simulink model "Inverter3P_VoltageControl_PI_s"  (R2024a)
settings: Solver=ode23tb  StartTime=0.0  StopTime=0.6  RelTol=1e-4
undefined symbols (not defined in the file): Cf, kii, kiv, kpi, kpv, Lf, rL, Rload_dm
libraries: spsSeriesRLCBranchLib x12, spsCurrentMeasurementLib x6, spsIGBTDiodeLib x6, spsVoltageMeasurementLib x4, spsIdealSwitchLib x3, spsDCVoltageSourceLib x1, spsPower3phPhasorLib x1, sps_lib x1
Description:
  | Copyright 2008 The MathWorks(TM), Inc.
settings Model: Creator=patrice  LastModifiedBy=ducnv
settings SolverCC: AlgebraicLoopSolver=TrustRegion
settings DataIOCC: SaveFormat=Array  SignalLoggingSaveFormat=ModelDataLogs  ReturnWorkspaceOutputs=off  SignalLoggingName=sigsOut
settings OptimizationCC: BlockReduction=off  BooleanDataType=off  ExpressionDepthLimit=2147483647  InitFltsAndDblsToZero=on  EfficientMapNaN2IntZero=off  LifeSpan=inf
settings DebuggingCC: UnderspecifiedInitializationDetection=Classic  MergeDetectMultiDrivingBlocksExec=none  CheckExecutionContextPreStartOutputMsg=on  SignalResolutionControl=TryResolveAllWithWarning  MultiTaskDSMMsg=warning  MultiTaskCondExecSysMsg=none  SigSpecEnsureSampleTimeMsg=none  FcnCallInpInsideContextMsg=warning  UnconnectedInputMsg=warning  UnconnectedOutputMsg=warning  UnconnectedLineMsg=warning  StateNameClashWarn=warning  SFUnexpectedBacktrackingDiag=warning  SFNoUnconditionalDefaultTransitionDiag=warning  SFExecutionAtInitializationDiag=none  ArithmeticOperatorsInVariantConditions=warning
settings HardwareCC: ProdBitPerPointer=32  ProdBitPerSizeT=32  ProdBitPerPtrDiffT=32  ProdLargestAtomicFloat=None  ProdIntDivRoundTo=Undefined  ProdEndianess=Unspecified  ProdWordSize=32  ProdHWDeviceType=32-bit Generic  TargetUnknown=on
settings ModelReferenceCC: PropagateSignalLabelsOutOfModel=off
settings SFSimCC: SimUseLocalCustomCode=off  CustomCodeUndefinedFunction=UseInterfaceOnly
settings RTWCC: RTWUseLocalCustomCode=off  GPUComputeCapability=3.5
settings CodeAppCC: StateflowObjectComments=on
settings GRTTargetCC: TargetLangStandard=C89/C90 (ANSI)  CombineOutputUpdateFcns=off  GRTInterface=on
settings ConfigComp: CovMetricSettings=dw  CovSaveCumulativeToWorkspaceVar=on  CovSaveSingleToWorkspaceVar=on  CovExternalEMLEnable=off
settings SimscapeCC: SimscapeNormalizeSystem=off

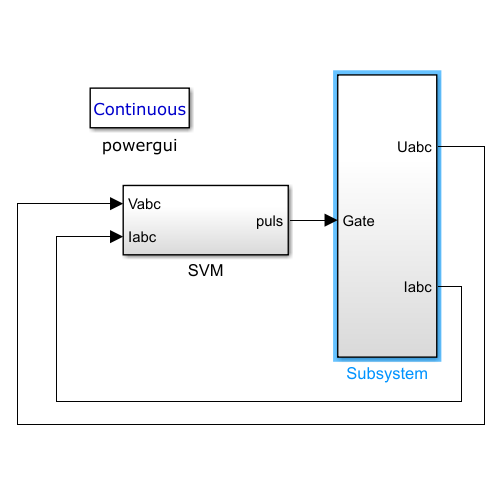
[thumbnail: Simulink's stored preview of the top-level diagram]
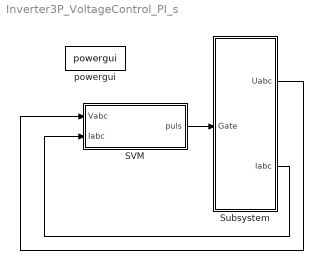
== system Inverter3P_VoltageControl_PI_s ==
  SVM : Subsystem
  Subsystem : Subsystem
  powergui : sps_lib/powergui  SimulationMode=Continuous  SampleTime=200e-6  frequency=60  Iterations=50  frequencyindice=0  Pbase=100e6  ErrMax=1e-4  UnitsV=kV  UnitsW=MW  buscounter=0  FunctionMessages=off  echomessages=off  EnableUseOfTLC=off  CurrentSourceSwitches=on  DisableSnubberDevices=off  DisableRonSwitches=off  DisableVfSwitches=off  DisplayEquations=off  AutomaticDiscreteSolvers=off  SolverType=Tustin  Interpol=off  ExternalGateDelay=off  methode=off  Ts=0  x0status=blocks  SPID=off  SwTol=0  HookPort=off  NonlinearTolerance=1e-4  nMaxIteration=100  ContinueOnMaxIteration=off  RestoreLinks=warning  ResistiveCurrentMeasurement=off  Frange=[0:2:500]  Ylog=off  Xlog=on  ShowGrid=off  save=off  variable=ZData  structure=ScopeData  ZoomFFT=off  StartTime=0.02  cycles=2  DisplayStyle=1  fundamental=50  FreqAxis=on  MaxFrequency=20000  frequencyindicesteady=1  RmsSteady=1  display=off
  wires:
  SVM/1(puls) -> Subsystem/1(Gate)
  Subsystem/2(Iabc) -> SVM/2(Iabc)
  Subsystem/1(Uabc) -> SVM/1(Vabc)

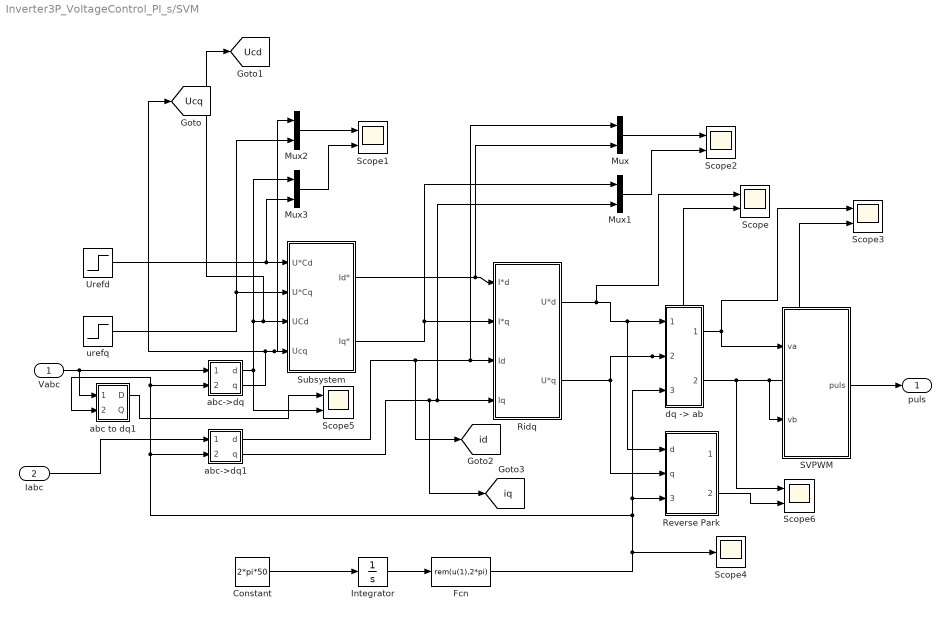
== system Inverter3P_VoltageControl_PI_s/SVM ==
  Vabc : Inport
  Iabc : Inport  Port=2
  Constant : Constant  Value=2*pi*50
  Fcn : Fcn  Expr=rem(u(1),2*pi)
  Integrator : Integrator
  Mux{,1..3} (4 alike) : Mux  Inputs=2
  Reverse Park : Subsystem
  Ridq : Subsystem
  SVPWM : Subsystem
  Scope{,1..3,5..6} (6 alike) : Scope  NumInputPorts=2
  Scope4 : Scope
  Subsystem : Subsystem
  Urefd : Step  Time=0  After=100  SampleTime=0
  abc to dq1 : Subsystem
  abc->dq : Subsystem  AncestorBlock=plecslib_extras/Transformations/3ph->RRF  mask(Transformation 3ph->RRF){}
      mask help:
      | Transforms a three-phase signal into a two-dimensional vector in a rotating reference frame. The rotation angle in radians of the rotating reference frame is determined by the second input:
      | [a b c], phi -> [d q]
      mask Help: web(['file://' plecsdoc '/abc2dq.html'])
      mask Display: plot([0 100],[0 100], [0.5 3 4 4 5 4 3 1 0 0 1 4]*4,[7 7 6 3 2 3 2 2 3 4 5 5]*4+62, [0 1 3 4 4 3 1 0 0 0]*4+24,[6 7 7 6 3 2 2 3 2 10]*4+62, [4 3 1 0 0 1 3 4]*4+48,[6 7 7 6 3 2 2 3]*4+62, [4 3 1 0 0 1 3 4 4 4]*4+52,[6 7 7 6 3 2 2 3 2 10]*4+5, [4 3 1 0 0 1 3 4 4 4]*4+76,[3 2 2 3 6 7 7 6 7 0]*4+5 )
  abc->dq1 : Subsystem  AncestorBlock=plecslib_extras/Transformations/3ph->RRF  mask(Transformation 3ph->RRF){}
      mask help:
      | Transforms a three-phase signal into a two-dimensional vector in a rotating reference frame. The rotation angle in radians of the rotating reference frame is determined by the second input:
      | [a b c], phi -> [d q]
      mask Help: web(['file://' plecsdoc '/abc2dq.html'])
      mask Display: plot([0 100],[0 100], [0.5 3 4 4 5 4 3 1 0 0 1 4]*4,[7 7 6 3 2 3 2 2 3 4 5 5]*4+62, [0 1 3 4 4 3 1 0 0 0]*4+24,[6 7 7 6 3 2 2 3 2 10]*4+62, [4 3 1 0 0 1 3 4]*4+48,[6 7 7 6 3 2 2 3]*4+62, [4 3 1 0 0 1 3 4 4 4]*4+52,[6 7 7 6 3 2 2 3 2 10]*4+5, [4 3 1 0 0 1 3 4 4 4]*4+76,[3 2 2 3 6 7 7 6 7 0]*4+5 )
  "dq -> ab" : Subsystem  mask(Coordinate converter){}
      mask help: The block converts 2 voltage (or rotor current , magnetic flux...) components which locate in rotor flux coordinate into 2 components located in fixed stator coordinate.The real axises of two coordinate locate askew each other an angle specified by the third input . The block has no parameters.
      mask Display:
      | plot([0 1],[0 1]);
      | text(0.3,0.7,'dq');text(0.7,0.4,'ab');
  urefq : Step  Time=0  After=sqrt(((220*sqrt(2))^2)-100^2)  SampleTime=0
  puls : Outport
  tag scope: Ucd=global, Ucq=global, id=global, iq=global
  wires:
  "dq -> ab"/1(Out1) -> Scope3/1, SVPWM/1(va)
  "dq -> ab"/2(Out2) -> Scope6/1, Scope3/2, SVPWM/2(vb)
  SVPWM/1(puls) -> puls/1
  Constant/1 -> Integrator/1
  Integrator/1 -> Fcn/1
  Ridq/1(U*d) -> Scope/1, Reverse Park/1(d), "dq -> ab"/1(In1)
  Ridq/2(U*q) -> Reverse Park/2(q), Scope/2, "dq -> ab"/2(In2)
  Urefd/1 -> Mux3/2, Subsystem/1(U*Cd)
  urefq/1 -> Mux2/2, Subsystem/2(U*Cq)
  abc->dq/1(d) -> Scope5/2, Mux3/1, [Ucd], Subsystem/3(UCd)
  abc->dq/2(q) -> [Ucq], Mux2/1, Subsystem/4(Ucq)
  abc->dq1/1(d) -> [id], Mux/1, Ridq/3(Id)
  abc->dq1/2(q) -> [iq], Mux1/2, Ridq/4(Iq)
  Vabc/1 -> abc to dq1/1(abc), abc->dq/1(abc)
  Iabc/1 -> abc->dq1/1(abc)
  Mux/1 -> Scope2/1
  Mux1/1 -> Scope2/2
  Mux2/1 -> Scope1/1
  Mux3/1 -> Scope1/2
  Fcn/1 -> Scope4/1, Reverse Park/3(Theta), "dq -> ab"/3(In3), abc->dq1/2(phi), abc to dq1/2(Theta), abc->dq/2(phi)
  abc to dq1/1(D) -> Scope5/1
  Reverse Park/2(Beta) -> Scope6/2
  Subsystem/1(Id*) -> Mux/2, Ridq/1(I*d)
  Subsystem/2(Iq*) -> Mux1/1, Ridq/2(I*q)

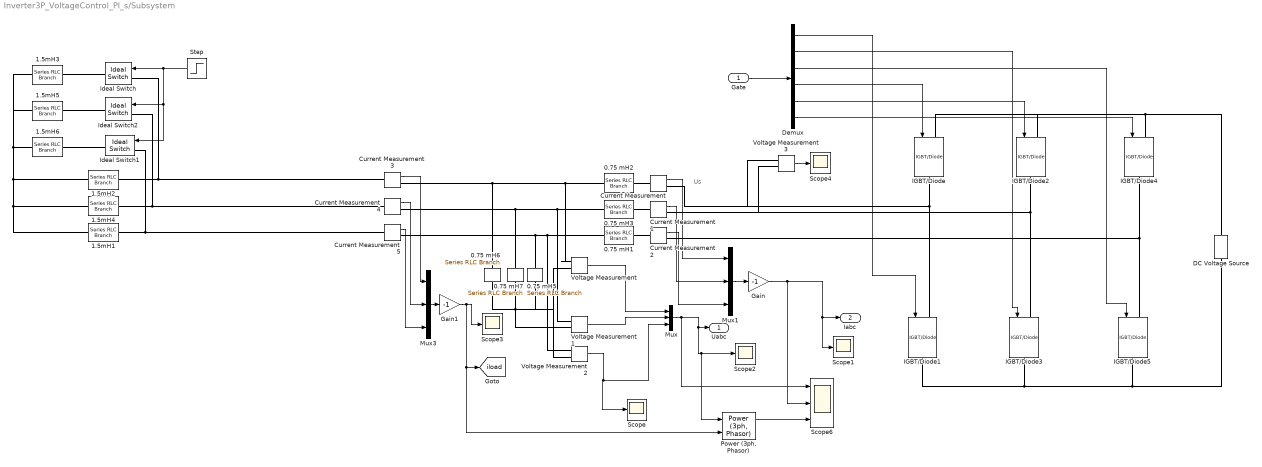
== system Inverter3P_VoltageControl_PI_s/Subsystem ==
  note: Us
  Gate : Inport
  0.75 mH1 : spsSeriesRLCBranchLib/Series RLC Branch  LConnTagsString=__new0  RConnTagsString=__new0  BranchType=RL  Resistance=rL  Inductance=Lf  SetiL0=off  InitialCurrent=0  Capacitance=1.0  Setx0=off  InitialVoltage=0  Measurements=None
  0.75 mH2 : spsSeriesRLCBranchLib/Series RLC Branch  LConnTagsString=__new0  RConnTagsString=__new0  BranchType=RL  Resistance=rL  Inductance=Lf  SetiL0=off  InitialCurrent=0  Capacitance=1.0  Setx0=off  InitialVoltage=0  Measurements=None
  0.75 mH3 : spsSeriesRLCBranchLib/Series RLC Branch  LConnTagsString=__new0  RConnTagsString=__new0  BranchType=RL  Resistance=rL  Inductance=Lf  SetiL0=off  InitialCurrent=0  Capacitance=1.0  Setx0=off  InitialVoltage=0  Measurements=None
  0.75 mH5 : spsSeriesRLCBranchLib/Series RLC Branch  LConnTagsString=__new0  RConnTagsString=__new0  BranchType=C  Resistance=1.0  Inductance=0.75e-3  SetiL0=off  InitialCurrent=0  Capacitance=Cf  Setx0=off  InitialVoltage=0  Measurements=None
  0.75 mH6 : spsSeriesRLCBranchLib/Series RLC Branch  LConnTagsString=__new0  RConnTagsString=__new0  BranchType=C  Resistance=1.0  Inductance=0.75e-3  SetiL0=off  InitialCurrent=0  Capacitance=Cf  Setx0=off  InitialVoltage=0  Measurements=None
  0.75 mH7 : spsSeriesRLCBranchLib/Series RLC Branch  LConnTagsString=__new0  RConnTagsString=__new0  BranchType=C  Resistance=1.0  Inductance=0.75e-3  SetiL0=off  InitialCurrent=0  Capacitance=Cf  Setx0=off  InitialVoltage=0  Measurements=None
  1.5mH{1..6} (6 alike) : spsSeriesRLCBranchLib/Series RLC Branch  LConnTagsString=__new0  RConnTagsString=__new0  BranchType=R  Resistance=Rload_dm*1.5  Inductance=2e-3  SetiL0=off  InitialCurrent=0  Capacitance=1.0  Setx0=off  InitialVoltage=0  Measurements=None
  Current Measurement{,1..5} (6 alike) : spsCurrentMeasurementLib/Current Measurement  PhasorSimulation=off  OutputType=Complex  PSBequivalent=0
  DC Voltage Source : spsDCVoltageSourceLib/DC Voltage Source  Amplitude=600  Measurements=None
  Demux : Demux  Outputs=6
  Gain : Gain  Gain=-1
  Gain1 : Gain  Gain=-1
  IGBT/Diode{,1..5} (6 alike) : spsIGBTDiodeLib/IGBT//Diode  Ron=1e-3  Rs=1e5  Cs=inf  Measurements=off
  Ideal Switch : spsIdealSwitchLib/Ideal Switch  Ron=0.001  Lon=0  IC=0  Rs=1e5  Cs=inf  Measurements=off
  Ideal Switch1 : spsIdealSwitchLib/Ideal Switch  Ron=0.001  Lon=0  IC=0  Rs=1e5  Cs=inf  Measurements=off
  Ideal Switch2 : spsIdealSwitchLib/Ideal Switch  Ron=0.001  Lon=0  IC=0  Rs=1e5  Cs=inf  Measurements=off
  Mux : Mux  Inputs=3
  Mux1 : Mux  Inputs=3
  Mux3 : Mux  Inputs=3
  "Power (3ph, Phasor)" : spsPower3phPhasorLib/Power (3ph, Phasor)
      settings: LibrarySourceBlock=|
      | sps_lib/Sensors and Measurements/Power
      | (3ph, Phasor)
  Scope{,1..4} (5 alike) : Scope
  Scope6 : Scope  NumInputPorts=3
  Step : Step  Time=0.3  SampleTime=0
  Voltage Measurement{,1..3} (4 alike) : spsVoltageMeasurementLib/Voltage Measurement  PhasorSimulation=off  OutputType=Complex  PSBequivalent=0
  Uabc : Outport
  Iabc : Outport  Port=2
  tag scope: iload=global
  wires:
  Gate/1 -> Demux/1
  Mux/1 -> Scope6/1, "Power (3ph, Phasor)"/1, Scope2/1, Uabc/1
  Mux1/1 -> Gain/1
  Gain/1 -> Scope6/2, Scope1/1, Iabc/1
  Voltage Measurement/1 -> Mux/1
  Voltage Measurement1/1 -> Mux/2
  Voltage Measurement2/1 -> Scope/1, Mux/3
  Current Measurement/1 -> Mux1/1
  Current Measurement1/1 -> Mux1/2
  Current Measurement2/1 -> Mux1/3
  Mux3/1 -> Gain1/1
  Gain1/1 -> [iload], "Power (3ph, Phasor)"/2, Scope3/1
  Current Measurement3/1 -> Mux3/1
  Current Measurement4/1 -> Mux3/2
  Current Measurement5/1 -> Mux3/3
  Voltage Measurement3/1 -> Scope4/1
  Demux/1 -> IGBT/Diode1/1
  Demux/2 -> IGBT/Diode3/1
  Demux/3 -> IGBT/Diode5/1
  Demux/4 -> IGBT/Diode/1
  Demux/5 -> IGBT/Diode2/1
  Demux/6 -> IGBT/Diode4/1
  Step/1 -> Ideal Switch1/1, Ideal Switch2/1, Ideal Switch/1
  "Power (3ph, Phasor)"/1 -> Scope6/3
  connections:
  IGBT/Diode2/LConn1 -- IGBT/Diode/LConn1 -- IGBT/Diode4/LConn1 -- DC Voltage Source/RConn1
  IGBT/Diode5/RConn1 -- IGBT/Diode1/RConn1 -- IGBT/Diode3/RConn1 -- DC Voltage Source/LConn1
  IGBT/Diode2/RConn1 -- Voltage Measurement3/LConn2 -- Current Measurement1/RConn1 -- IGBT/Diode3/LConn1
  IGBT/Diode5/LConn1 -- Current Measurement2/RConn1 -- IGBT/Diode4/RConn1
  IGBT/Diode/RConn1 -- Voltage Measurement3/LConn1 -- Current Measurement/RConn1 -- IGBT/Diode1/LConn1
  0.75 mH5/RConn1 -- Current Measurement5/RConn1 -- 0.75 mH1/LConn1 -- Voltage Measurement2/LConn1
  0.75 mH7/RConn1 -- Current Measurement4/RConn1 -- 0.75 mH3/LConn1 -- Voltage Measurement1/LConn1
  0.75 mH6/RConn1 -- Current Measurement3/RConn1 -- Voltage Measurement/LConn1 -- 0.75 mH2/LConn1
  0.75 mH2/RConn1 -- Current Measurement/LConn1
  0.75 mH3/RConn1 -- Current Measurement1/LConn1
  0.75 mH1/RConn1 -- Current Measurement2/LConn1
  0.75 mH6/LConn1 -- Voltage Measurement/LConn2 -- Voltage Measurement2/LConn2 -- Voltage Measurement1/LConn2 -- 0.75 mH7/LConn1 -- 0.75 mH5/LConn1
  Ideal Switch/LConn1 -- Current Measurement3/LConn1 -- 1.5mH2/LConn1
  Current Measurement5/LConn1 -- Ideal Switch1/LConn1 -- 1.5mH1/LConn1
  Current Measurement4/LConn1 -- Ideal Switch2/LConn1 -- 1.5mH4/LConn1
  1.5mH2/RConn1 -- 1.5mH3/RConn1 -- 1.5mH5/RConn1 -- 1.5mH6/RConn1 -- 1.5mH1/RConn1 -- 1.5mH4/RConn1
  1.5mH6/LConn1 -- Ideal Switch1/RConn1
  1.5mH5/LConn1 -- Ideal Switch2/RConn1
  1.5mH3/LConn1 -- Ideal Switch/RConn1

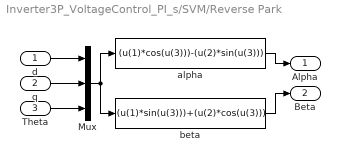
== system Inverter3P_VoltageControl_PI_s/SVM/Reverse Park ==
  d : Inport
  q : Inport  Port=2
  Theta : Inport  Port=3
  Mux : Mux  Inputs=3
  alpha : Fcn  Expr=(u(1)*cos(u(3)))-(u(2)*sin(u(3)))
  beta : Fcn  Expr=(u(1)*sin(u(3)))+(u(2)*cos(u(3)))
  Alpha : Outport  VectorParamsAs1DForOutWhenUnconnected=off
  Beta : Outport  Port=2  VectorParamsAs1DForOutWhenUnconnected=off
  wires:
  alpha/1 -> Alpha/1
  beta/1 -> Beta/1
  Mux/1 -> beta/1, alpha/1
  d/1 -> Mux/1
  q/1 -> Mux/2
  Theta/1 -> Mux/3

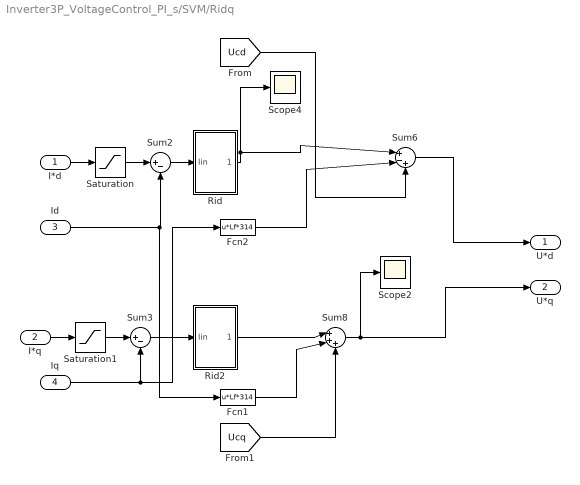
== system Inverter3P_VoltageControl_PI_s/SVM/Ridq ==
  I*d : Inport
  I*q : Inport  Port=2
  Id : Inport  Port=3
  Iq : Inport  Port=4
  Fcn1 : Fcn  Expr=u*Lf*314
  Fcn2 : Fcn  Expr=u*Lf*314
  Rid : Subsystem
  Rid2 : Subsystem
  Saturation : Saturate  UpperLimit=15.15*sqrt(2)
  Saturation1 : Saturate  UpperLimit=15.15*sqrt(2)
  Scope2 : Scope
  Scope4 : Scope
  Sum2 : Sum  Inputs=|+-
  Sum3 : Sum  Inputs=|+-
  Sum6 : Sum  Inputs=|+-+
  Sum8 : Sum  Inputs=|+++
  U*d : Outport
  U*q : Outport  Port=2
  wires:
  Id/1 -> Fcn1/1, Sum2/2
  I*d/1 -> Saturation/1
  I*q/1 -> Saturation1/1
  Fcn1/1 -> Sum8/2
  Fcn2/1 -> Sum6/2
  Sum3/1 -> Rid2/1(Iin)
  Sum2/1 -> Rid/1(Iin)
  Iq/1 -> Fcn2/1, Sum3/2
  Sum8/1 -> Scope2/1, U*q/1
  Sum6/1 -> U*d/1
  [Ucq] -> Sum8/3
  [Ucd] -> Sum6/3
  Rid/1(dUL) -> Sum6/1, Scope4/1
  Rid2/1(dUL) -> Sum8/1
  Saturation/1 -> Sum2/1
  Saturation1/1 -> Sum3/1

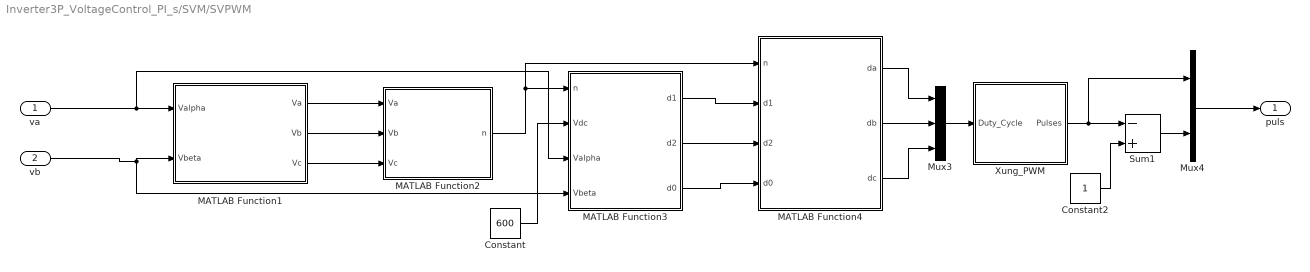
== system Inverter3P_VoltageControl_PI_s/SVM/SVPWM ==
  va : Inport
  vb : Inport  Port=2
  Constant : Constant  Value=600
  Constant2 : Constant
  MATLAB Function1 : MATLAB Function  TreatAsAtomicUnit=on
  MATLAB Function2 : MATLAB Function  TreatAsAtomicUnit=on
  MATLAB Function3 : MATLAB Function  TreatAsAtomicUnit=on
  MATLAB Function4 : MATLAB Function  TreatAsAtomicUnit=on
  Mux3 : Mux  Inputs=3
  Mux4 : Mux  Inputs=2
  Sum1 : Sum  Inputs=-+
  Xung_PWM : Subsystem
  puls : Outport
  wires:
  Constant/1 -> MATLAB Function3/2(Vdc)
  MATLAB Function1/3(Vc) -> MATLAB Function2/3(Vc)
  MATLAB Function1/2(Vb) -> MATLAB Function2/2(Vb)
  Mux4/1 -> puls/1
  Sum1/1 -> Mux4/2
  Xung_PWM/1(Pulses) -> Mux4/1, Sum1/1
  MATLAB Function2/1(n) -> MATLAB Function4/1(n), MATLAB Function3/1(n)
  Mux3/1 -> Xung_PWM/1(Duty_Cycle)
  vb/1 -> MATLAB Function3/4(Vbeta), MATLAB Function1/2(Vbeta)
  MATLAB Function3/3(d0) -> MATLAB Function4/4(d0)
  MATLAB Function3/1(d1) -> MATLAB Function4/2(d1)
  MATLAB Function4/1(da) -> Mux3/1
  MATLAB Function1/1(Va) -> MATLAB Function2/1(Va)
  MATLAB Function4/3(dc) -> Mux3/3
  MATLAB Function3/2(d2) -> MATLAB Function4/3(d2)
  MATLAB Function4/2(db) -> Mux3/2
  va/1 -> MATLAB Function3/3(Valpha), MATLAB Function1/1(Valpha)
  Constant2/1 -> Sum1/2

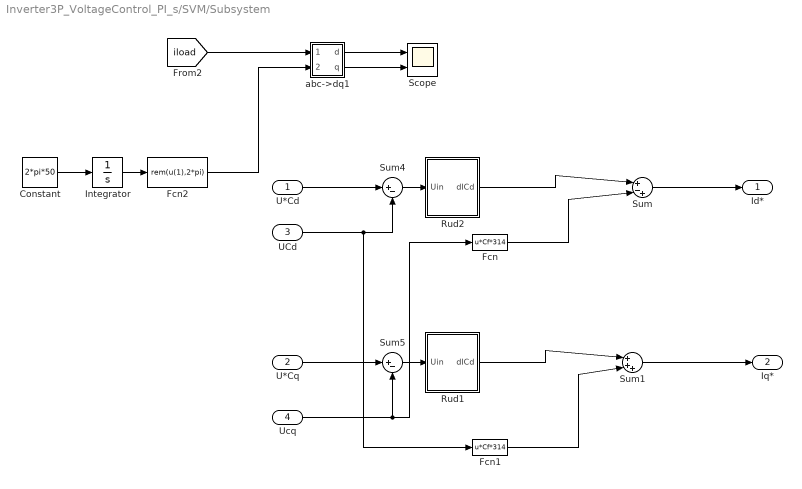
== system Inverter3P_VoltageControl_PI_s/SVM/Subsystem ==
  U*Cd : Inport
  U*Cq : Inport  Port=2
  UCd : Inport  Port=3
  Ucq : Inport  Port=4
  Constant : Constant  Value=2*pi*50
  Fcn : Fcn  Expr=u*Cf*314
  Fcn1 : Fcn  Expr=u*Cf*314
  Fcn2 : Fcn  Expr=rem(u(1),2*pi)
  Integrator : Integrator
  Rud1 : Subsystem
  Rud2 : Subsystem
  Scope : Scope  NumInputPorts=2
  Sum : Sum  Inputs=|+-+
  Sum1 : Sum  Inputs=|+++
  Sum4 : Sum  Inputs=|+-
  Sum5 : Sum  Inputs=|+-
  abc->dq1 : Subsystem  AncestorBlock=plecslib_extras/Transformations/3ph->RRF  mask(Transformation 3ph->RRF){}
      mask help:
      | Transforms a three-phase signal into a two-dimensional vector in a rotating reference frame. The rotation angle in radians of the rotating reference frame is determined by the second input:
      | [a b c], phi -> [d q]
      mask Help: web(['file://' plecsdoc '/abc2dq.html'])
      mask Display: plot([0 100],[0 100], [0.5 3 4 4 5 4 3 1 0 0 1 4]*4,[7 7 6 3 2 3 2 2 3 4 5 5]*4+62, [0 1 3 4 4 3 1 0 0 0]*4+24,[6 7 7 6 3 2 2 3 2 10]*4+62, [4 3 1 0 0 1 3 4]*4+48,[6 7 7 6 3 2 2 3]*4+62, [4 3 1 0 0 1 3 4 4 4]*4+52,[6 7 7 6 3 2 2 3 2 10]*4+5, [4 3 1 0 0 1 3 4 4 4]*4+76,[3 2 2 3 6 7 7 6 7 0]*4+5 )
  Id* : Outport
  Iq* : Outport  Port=2
  wires:
  Sum/1 -> Id*/1
  Sum1/1 -> Iq*/1
  UCd/1 -> Fcn1/1, Sum4/2
  Ucq/1 -> Fcn/1, Sum5/2
  U*Cq/1 -> Sum5/1
  Rud1/1(dICd) -> Sum1/1
  Rud2/1(dICd) -> Sum/1
  Sum4/1 -> Rud2/1(Uin)
  Fcn1/1 -> Sum1/2
  Sum5/1 -> Rud1/1(Uin)
  Fcn/1 -> Sum/2
  U*Cd/1 -> Sum4/1
  [iload] -> abc->dq1/1(abc)
  Integrator/1 -> Fcn2/1
  Constant/1 -> Integrator/1
  Fcn2/1 -> abc->dq1/2(phi)
  abc->dq1/1(d) -> Scope/1
  abc->dq1/2(q) -> Scope/2

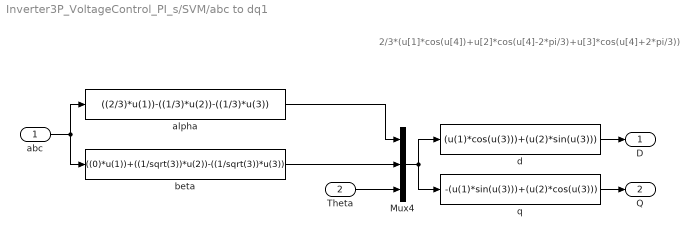
== system Inverter3P_VoltageControl_PI_s/SVM/abc to dq1 ==
  note: 2/3*(u[1]*cos(u[4])+u[2]*cos(u[4]-2*pi/3)+u[3]*cos(u[4]+2*pi/3))
  abc : Inport
  Theta : Inport  Port=2
  Mux4 : Mux  Inputs=3
  alpha : Fcn  Expr=((2/3)*u(1))-((1/3)*u(2))-((1/3)*u(3))
  beta : Fcn  Expr=((0)*u(1))+((1/sqrt(3))*u(2))-((1/sqrt(3))*u(3))
  d : Fcn  Expr=(u(1)*cos(u(3)))+(u(2)*sin(u(3)))
  q : Fcn  Expr=-(u(1)*sin(u(3)))+(u(2)*cos(u(3)))
  D : Outport  VectorParamsAs1DForOutWhenUnconnected=off
  Q : Outport  Port=2  VectorParamsAs1DForOutWhenUnconnected=off
  wires:
  Theta/1 -> Mux4/3
  q/1 -> Q/1
  alpha/1 -> Mux4/1
  d/1 -> D/1
  beta/1 -> Mux4/2
  abc/1 -> alpha/1, beta/1
  Mux4/1 -> d/1, q/1

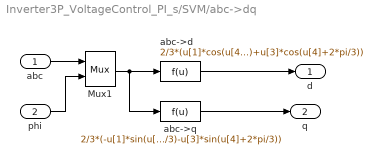
== system Inverter3P_VoltageControl_PI_s/SVM/abc->dq ==
  abc : Inport  PortDimensions=3
  phi : Inport  Port=2  PortDimensions=1
  Mux1 : Mux  Inputs=2
  abc->d : Fcn  Expr=2/3*(u[1]*cos(u[4])+u[2]*cos(u[4]-2*pi/3)+u[3]*cos(u[4]+2*pi/3))
  abc->q : Fcn  Expr=2/3*(-u[1]*sin(u[4])-u[2]*sin(u[4]-2*pi/3)-u[3]*sin(u[4]+2*pi/3))
  d : Outport
  q : Outport  Port=2
  wires:
  Mux1/1 -> abc->d/1, abc->q/1
  abc->q/1 -> q/1
  abc->d/1 -> d/1
  abc/1 -> Mux1/1
  phi/1 -> Mux1/2

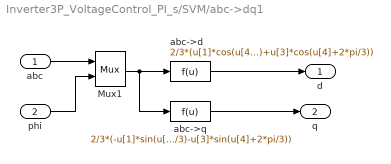
== system Inverter3P_VoltageControl_PI_s/SVM/abc->dq1 ==
  abc : Inport  PortDimensions=3
  phi : Inport  Port=2  PortDimensions=1
  Mux1 : Mux  Inputs=2
  abc->d : Fcn  Expr=2/3*(u[1]*cos(u[4])+u[2]*cos(u[4]-2*pi/3)+u[3]*cos(u[4]+2*pi/3))
  abc->q : Fcn  Expr=2/3*(-u[1]*sin(u[4])-u[2]*sin(u[4]-2*pi/3)-u[3]*sin(u[4]+2*pi/3))
  d : Outport
  q : Outport  Port=2
  wires:
  phi/1 -> Mux1/2
  abc/1 -> Mux1/1
  abc->d/1 -> d/1
  abc->q/1 -> q/1
  Mux1/1 -> abc->q/1, abc->d/1

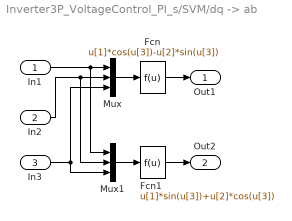
== system Inverter3P_VoltageControl_PI_s/SVM/dq -> ab ==
  In1 : Inport
  In2 : Inport  Port=2
  In3 : Inport  Port=3
  Fcn : Fcn  Expr=u[1]*cos(u[3])-u[2]*sin(u[3])
  Fcn1 : Fcn  Expr=u[1]*sin(u[3])+u[2]*cos(u[3])
  Mux : Mux  Inputs=3
  Mux1 : Mux  Inputs=3
  Out1 : Outport  InitialOutput=0
  Out2 : Outport  Port=2  InitialOutput=0
  wires:
  In1/1 -> Mux/1, Mux1/1
  In2/1 -> Mux/2, Mux1/2
  In3/1 -> Mux/3, Mux1/3
  Mux/1 -> Fcn/1
  Mux1/1 -> Fcn1/1
  Fcn/1 -> Out1/1
  Fcn1/1 -> Out2/1

== system Inverter3P_VoltageControl_PI_s/SVM/Ridq/Rid ==
  Iin : Inport
  Gain : Gain  Gain=kii
  Gain1 : Gain  Gain=kpi
  Integrator : Integrator
  Sum : Sum  Inputs=|++
  dUL : Outport
  wires:
  Sum/1 -> dUL/1
  Integrator/1 -> Sum/2
  Gain1/1 -> Sum/1
  Gain/1 -> Integrator/1
  Iin/1 -> Gain/1, Gain1/1

== system Inverter3P_VoltageControl_PI_s/SVM/Ridq/Rid2 ==
  Iin : Inport
  Gain : Gain  Gain=kii
  Gain1 : Gain  Gain=kpi
  Integrator : Integrator
  Sum : Sum  Inputs=|++
  dUL : Outport
  wires:
  Sum/1 -> dUL/1
  Integrator/1 -> Sum/2
  Gain1/1 -> Sum/1
  Gain/1 -> Integrator/1
  Iin/1 -> Gain/1, Gain1/1

== system Inverter3P_VoltageControl_PI_s/SVM/SVPWM/Xung_PWM ==
  Duty_Cycle : Inport
  Relay : Relay
  Sawtooth : Subsystem
  Scope : Scope
  Sum4 : Sum  Inputs=-+|  InputSameDT=on  SaturateOnIntegerOverflow=on  OutDataTypeStr=Inherit: Same as first input
  Pulses : Outport  VectorParamsAs1DForOutWhenUnconnected=off
  wires:
  Sum4/1 -> Relay/1
  Duty_Cycle/1 -> Sum4/2
  Sawtooth/1(Pulses) -> Scope/1, Sum4/1
  Relay/1 -> Pulses/1

== system Inverter3P_VoltageControl_PI_s/SVM/Subsystem/Rud1 ==
  Uin : Inport
  Gain : Gain  Gain=kiv
  Gain1 : Gain  Gain=kpv
  Integrator : Integrator
  Sum : Sum  Inputs=|++
  dICd : Outport
  wires:
  Integrator/1 -> Sum/2
  Uin/1 -> Gain1/1, Gain/1
  Gain1/1 -> Sum/1
  Gain/1 -> Integrator/1
  Sum/1 -> dICd/1

== system Inverter3P_VoltageControl_PI_s/SVM/Subsystem/Rud2 ==
  Uin : Inport
  Gain : Gain  Gain=kiv
  Gain1 : Gain  Gain=kpv
  Integrator : Integrator
  Sum : Sum  Inputs=|++
  dICd : Outport
  wires:
  Integrator/1 -> Sum/2
  Uin/1 -> Gain1/1, Gain/1
  Gain1/1 -> Sum/1
  Gain/1 -> Integrator/1
  Sum/1 -> dICd/1

== system Inverter3P_VoltageControl_PI_s/SVM/Subsystem/abc->dq1 ==
  abc : Inport  PortDimensions=3
  phi : Inport  Port=2  PortDimensions=1
  Mux1 : Mux  Inputs=2
  abc->d : Fcn  Expr=2/3*(u[1]*cos(u[4])+u[2]*cos(u[4]-2*pi/3)+u[3]*cos(u[4]+2*pi/3))
  abc->q : Fcn  Expr=2/3*(-u[1]*sin(u[4])-u[2]*sin(u[4]-2*pi/3)-u[3]*sin(u[4]+2*pi/3))
  d : Outport
  q : Outport  Port=2
  wires:
  phi/1 -> Mux1/2
  abc/1 -> Mux1/1
  abc->d/1 -> d/1
  abc->q/1 -> q/1
  Mux1/1 -> abc->q/1, abc->d/1

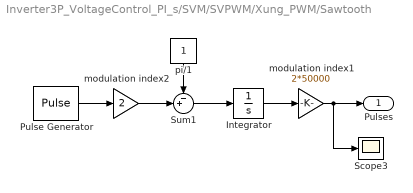
== system Inverter3P_VoltageControl_PI_s/SVM/SVPWM/Xung_PWM/Sawtooth ==
  Integrator : Integrator
  Pulse Generator : DiscretePulseGenerator  PulseType=Time based  Period=1/50000  PulseWidth=50
  Scope3 : Scope
  Sum1 : Sum  Inputs=-+|  InputSameDT=on  SaturateOnIntegerOverflow=on  OutDataTypeStr=Inherit: Same as first input
  modulation index1 : Gain  Gain=2*50000  SaturateOnIntegerOverflow=on  OutDataTypeStr=Inherit: Same as input  ParamDataTypeStr=Inherit: Same as input
  modulation index2 : Gain  Gain=2  SaturateOnIntegerOverflow=on  OutDataTypeStr=Inherit: Same as input  ParamDataTypeStr=Inherit: Same as input
  pi/1 : Constant
  Pulses : Outport  VectorParamsAs1DForOutWhenUnconnected=off
  wires:
  Pulse Generator/1 -> modulation index2/1
  Integrator/1 -> modulation index1/1
  modulation index1/1 -> Pulses/1, Scope3/1
  Sum1/1 -> Integrator/1
  modulation index2/1 -> Sum1/2
  pi/1/1 -> Sum1/1

== matlab function Inverter3P_VoltageControl_PI_s/SVM/SVPWM/MATLAB Function1 ==
  data: Valpha input; Va output; Vbeta input; Vb output; Vc output
function [Va,Vb,Vc] = Rev_Clark(Valpha,Vbeta)
Va = Valpha;
Vb = -Valpha/2 + sqrt(3)*Vbeta/2;
Vc = -Valpha/2 - sqrt(3)*Vbeta/2;

== matlab function Inverter3P_VoltageControl_PI_s/SVM/SVPWM/MATLAB Function2 ==
  data: Va input; n output; Vb input; Vc input
function n = Sector(Va,Vb,Vc)
n = 0;
if (Va >= Vb)
    if(Vb >= Vc)
        n = 1;
    else
        if (Vc >= Va)
            n = 5;
        else
            n = 6;
        end
    end
else
    if (Vb < Vc)
        n = 4;
    else
        if (Vc < Va)
            n = 2;
        else
            n = 3;
        end
    end
end

== matlab function Inverter3P_VoltageControl_PI_s/SVM/SVPWM/MATLAB Function3 ==
  data: n input; d1 output; Vdc input; Valpha input; Vbeta input; d2 output; d0 output
function [d1,d2,d0] = Duty(n,Vdc,Valpha,Vbeta)
d0 = 0;
d1 = 0;
d2 = 0;
if (n == 1)
    d1 = 1/Vdc*(3/2*Valpha - sqrt(3)/2*Vbeta);
    d2 = 1/Vdc*(0*Valpha + sqrt(3)*Vbeta);
    d0 = 1-d1-d2;
end
if (n == 2)
    d1 = 1/Vdc*(-3/2*Valpha + sqrt(3)/2*Vbeta);
    d2 = 1/Vdc*(3/2*Valpha + sqrt(3)/2*Vbeta);
    d0 = 1-d1-d2;
end
if (n == 3)
    d1 = 1/Vdc*(0*Valpha + sqrt(3)*Vbeta);
    d2 = 1/Vdc*(-3/2*Valpha - sqrt(3)/2*Vbeta);
    d0 = 1-d1-d2;
end
if (n == 4)
    d1 = 1/Vdc*(0*Valpha - sqrt(3)*Vbeta);
    d2 = 1/Vdc*(-3/2*Valpha + sqrt(3)/2*Vbeta);
    d0 = 1-d1-d2; 
end
if (n == 5)
    d1 = 1/Vdc*(-3/2*Valpha - sqrt(3)/2*Vbeta);
    d2 = 1/Vdc*(3/2*Valpha - sqrt(3)/2*Vbeta);
    d0 = 1-d1-d2;
end
if (n == 6)
    d1 = 1/Vdc*(3/2*Valpha + sqrt(3)/2*Vbeta);
    d2 = 1/Vdc*(0*Valpha - sqrt(3)*Vbeta);
    d0 = 1-d1-d2; 
end

== matlab function Inverter3P_VoltageControl_PI_s/SVM/SVPWM/MATLAB Function4 ==
  data: n input; da output; d1 input; d2 input; d0 input; db output; dc output
function [da,db,dc] = Duty_Cycle(n,d1,d2,d0)
da = 0;
db = 0;
dc = 0;
if (n == 1)
    da = d0/2;
    db = d0/2 + d1;
    dc = d0/2 + d1 + d2;
end
if (n == 2)
    da = d0/2 + d1;
    db = d0/2;
    dc = d0/2 + d1 + d2;
end
if (n == 3)
    da = d0/2 + d1 + d2;
    db = d0/2;
    dc = d0/2 + d1;
end
if (n == 4)
    da = d0/2 + d1 + d2;
    db = d0/2 + d1;
    dc = d0/2;
end
if (n == 5)
    da = d0/2 + d1;
    db = d0/2 + d1 + d2;
    dc = d0/2;
end
if (n == 6)
    da = d0/2;
    db = d0/2 + d1 + d2;
    dc = d0/2 + d1;
end
